simulink model "Decuplare_intrari_nec"  (R2020b)
settings: Solver=VariableStepAuto  StartTime=0.0  StopTime=1  RelTol=1e-3
values from neighbouring files (symbols this model uses):
  Ad = eye(size(A))+Ts*A    [Script_pendul.m]
  Bd = Ts*B    [Script_pendul.m]
  Cd = C    [Script_pendul.m]
  E = [0.5 0 0.1 0]'    [Script_pendul.m]
  F = T*Ad-K1*Cd    [Script_pendul.m]
  H = E*pinv(Cd*E)    [Script_pendul.m]
  K1 = K1'    [Script_pendul.m]
  K2 = F*H    [Script_pendul.m]
  T = eye(4)-H*Cd    [Script_pendul.m]
  Ts = 0.001    [Script_pendul.m]
libraries: eeStairGenerator x1
settings Model: Creator=tudor  LastModifiedBy=tudor

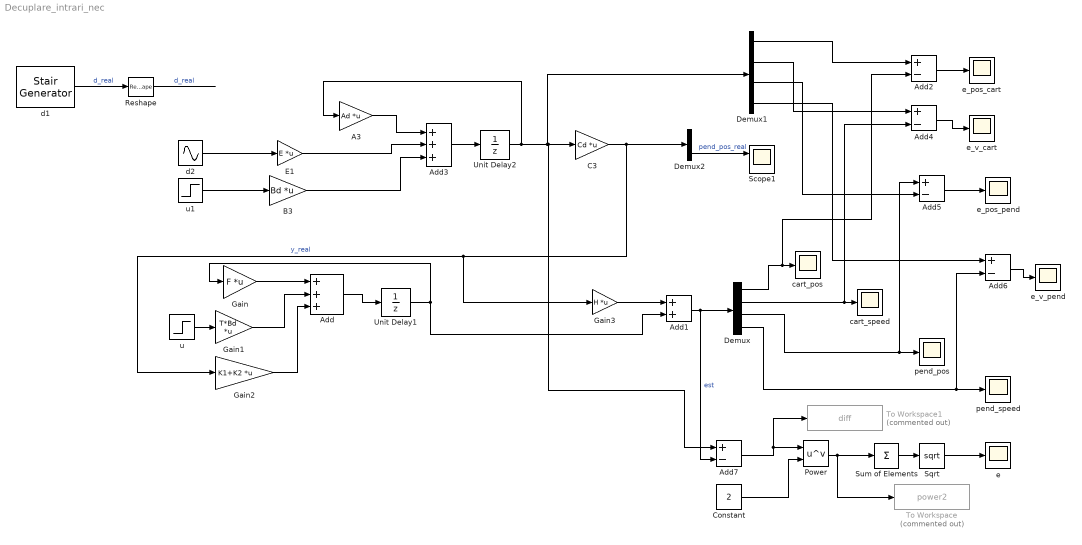
== system Decuplare_intrari_nec ==
  A3 : Gain  Gain=Ad  Multiplication=Matrix(K*u)
  Add : Sum  Inputs=+++
  Add1 : Sum
  Add{2,4..7} (5 alike) : Sum  Inputs=+-
  Add3 : Sum  Inputs=+++
  B3 : Gain  Gain=Bd  Multiplication=Matrix(K*u)
  C3 : Gain  Gain=Cd  Multiplication=Matrix(K*u)
  Constant : Constant  Value=2
  Demux : Demux
  Demux1 : Demux
  Demux2 : Demux  Outputs=2
  E1 : Gain  Gain=E  Multiplication=Matrix(K*u)
  Gain : Gain  Gain=F  Multiplication=Matrix(K*u)
  Gain1 : Gain  Gain=T*Bd  Multiplication=Matrix(K*u)
  Gain2 : Gain  Gain=K1+K2  Multiplication=Matrix(K*u)
  Gain3 : Gain  Gain=H  Multiplication=Matrix(K*u)
  Power : Math  Operator=pow  SaturateOnIntegerOverflow=on
  Reshape : Reshape
  Scope1 : Scope  NumInputPorts=2
  Sqrt : Sqrt  SaturateOnIntegerOverflow=on
  Sum of Elements : Sum  Inputs=+
  To Workspace : ToWorkspace  Commented=on  VariableName=power2  SampleTime=-1
  To Workspace1 : ToWorkspace  Commented=on  VariableName=diff  SampleTime=-1
  Unit Delay1 : UnitDelay  InitialCondition=[0 0 1 0]  SampleTime=Ts  HasFrameUpgradeWarning=on
  Unit Delay2 : UnitDelay  InitialCondition=[0 0 0 0]  SampleTime=Ts  HasFrameUpgradeWarning=on
  cart_pos : Scope
  cart_speed : Scope
  d1 : eeStairGenerator/Stair Generator  LabelModeActiveChoice=Discrete  TimeInput=[0 1 3]  AmplitudeInput=[0 0.1 -0.3]  SampleTime=Ts  RepeatPattern=off  OutDataTypeStr=double
      settings: SourceProductBaseCode=PS
  d2 : Sin  Amplitude=0.1  Frequency=20  SampleTime=Ts
  e : Scope
  e_pos_cart : Scope
  e_pos_pend : Scope
  e_v_cart : Scope
  e_v_pend : Scope
  pend_pos : Scope
  pend_speed : Scope
  u : Step  Time=0  After=0  SampleTime=Ts
  u1 : Step  Time=0  After=0  SampleTime=Ts
  wires:
  B3/1 -> Add3/3
  Unit Delay2/1 -> Add7/1, C3/1, Demux1/1, A3/1
  C3/1 -> Gain3/1, Gain2/1, Demux2/1  "y_real"
  Demux2/2 -> Scope1/1  "pend_pos_real"
  E1/1 -> Add3/2
  A3/1 -> Add3/1
  u1/1 -> B3/1
  Add3/1 -> Unit Delay2/1
  u/1 -> Gain1/1
  d2/1 -> E1/1
  Gain/1 -> Add/1
  Gain1/1 -> Add/2
  d1/1 -> Reshape/1  "d_real"
  Reshape/1 -> ?  "d_real"
  Gain2/1 -> Add/3
  Add/1 -> Unit Delay1/1
  Unit Delay1/1 -> Add1/2, Gain/1
  Gain3/1 -> Add1/1
  Add1/1 -> Add7/2, Demux/1  "est"
  Demux/1 -> Add2/2, cart_pos/1
  Demux/2 -> Add4/2, cart_speed/1
  Demux/3 -> Add5/1, pend_pos/1
  Demux/4 -> Add6/2, pend_speed/1
  Add2/1 -> e_pos_cart/1
  Demux1/1 -> Add2/1
  Demux1/2 -> Add4/1
  Demux1/3 -> Add5/2
  Add4/1 -> e_v_cart/1
  Add5/1 -> e_pos_pend/1
  Add6/1 -> e_v_pend/1
  Demux1/4 -> Add6/1
  Constant/1 -> Power/2
  Add7/1 -> To Workspace1/1, Power/1
  Sqrt/1 -> e/1
  Sum of Elements/1 -> Sqrt/1
  Power/1 -> To Workspace/1, Sum of Elements/1
